simulink model "Tire_road_interaction_model"  (R2024b)
settings: Solver=VariableStepAuto  StartTime=0.0  StopTime=10.0  RelTol=1e-3
settings Model: Creator=francescovalentia  LastModifiedBy=francescovalentia

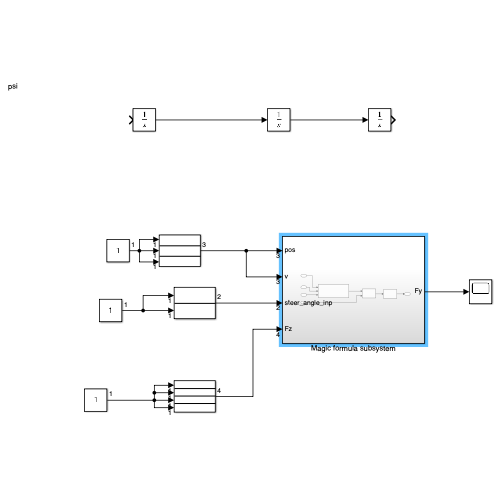
[thumbnail: Simulink's stored preview of the top-level diagram]
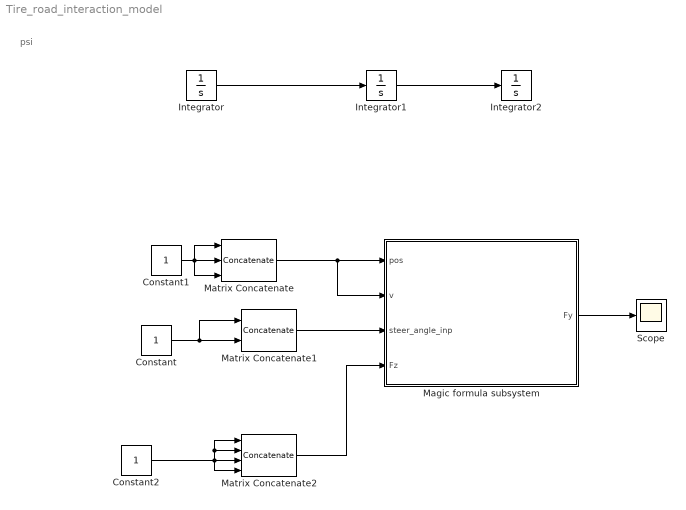
== system Tire_road_interaction_model ==
  note: psi
  Constant : Constant
  Constant1 : Constant
  Constant2 : Constant
  Integrator : Integrator
  Integrator1 : Integrator
  Integrator2 : Integrator
  Magic formula subsystem : Subsystem
  Matrix Concatenate : Concatenate  NumInputs=3  ConcatenateDimension=2
  Matrix Concatenate1 : Concatenate  ConcatenateDimension=2
  Matrix Concatenate2 : Concatenate  NumInputs=4  ConcatenateDimension=2
  Scope : Scope
  wires:
  Magic formula subsystem/1(Fy) -> Scope/1
  Constant1/1 -> Matrix Concatenate/2, Matrix Concatenate/3, Matrix Concatenate/1
  Matrix Concatenate/1 -> Magic formula subsystem/2(v), Magic formula subsystem/1(pos)
  Constant/1 -> Matrix Concatenate1/1, Matrix Concatenate1/2
  Matrix Concatenate1/1 -> Magic formula subsystem/3(steer_angle_inp)
  Constant2/1 -> Matrix Concatenate2/2, Matrix Concatenate2/1, Matrix Concatenate2/4, Matrix Concatenate2/3
  Matrix Concatenate2/1 -> Magic formula subsystem/4(Fz)
  Integrator/1 -> Integrator1/1
  Integrator1/1 -> Integrator2/1

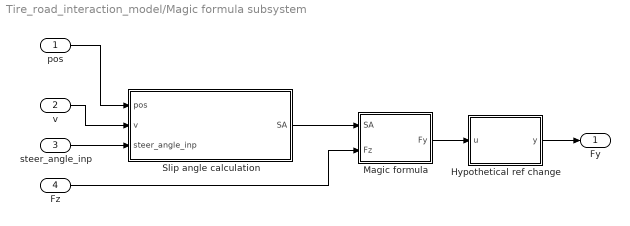
== system Tire_road_interaction_model/Magic formula subsystem ==
  pos : Inport
  v : Inport  Port=2
  steer_angle_inp : Inport  Port=3
  Fz : Inport  Port=4
  Hypothetical ref change : MATLAB Function  TreatAsAtomicUnit=on
  Magic formula : MATLAB Function  TreatAsAtomicUnit=on
  Slip angle calculation : MATLAB Function  TreatAsAtomicUnit=on
  Fy : Outport
  wires:
  Slip angle calculation/1(SA) -> Magic formula/1(SA)
  pos/1 -> Slip angle calculation/1(pos)
  Fz/1 -> Magic formula/2(Fz)
  v/1 -> Slip angle calculation/2(v)
  steer_angle_inp/1 -> Slip angle calculation/3(steer_angle_inp)
  Magic formula/1(Fy) -> Hypothetical ref change/1(u)
  Hypothetical ref change/1(y) -> Fy/1

== matlab function Tire_road_interaction_model/Magic formula subsystem/Slip angle calculation ==
  data: pos input; v input; SA output; steer_angle_inp input
function SA = fcn(pos, v, steer_angle_inp)
% pos = [xc, yc, psi]
% v = [xcdot; ycdot; psidot]
% steer_angle_inp = [left, right]
% r = distance between c and the wheel

r = 1; % distance between c and the wheels
alpha = 0;
v_complex = v(1) + 1j*v(2) + v(3) * r * exp(1j*(pi/2 + alpha + pos(3)));
v_angle = angle(v_complex);


SA = [v_angle - (pos(3) + steer_angle_inp(1)), v_angle - (pos(3) + steer_angle_inp(2)), v_angle - pos(3), v_angle - pos(3)]; % sign might be adjusted

== matlab function Tire_road_interaction_model/Magic formula subsystem/Hypothetical ref change ==
  data: u input; y output
function y = fcn(u)

y = u;

== matlab function Tire_road_interaction_model/Magic formula subsystem/Magic formula ==
  data: SA input; Fy output; Fz input
function Fy = fcn(SA, Fz)
% MAgic formula based on the data extracted from the TTC files



% influenc of the camber has to added !!!!


params = B1654run15_params.ForceY.P1.deg0;
Fy = Fz .*(params(3) * sin(params(2) * atan(params(1) * SA - params(4) * (params(1) * SA - atan(params(1) * SA)))));
